simulink model "SG_GFOR_2020a_REAL"  (R2020a)
settings: Solver=ode1  StartTime=0.0  StopTime=Tsim  FixedStep=Ts  MaxStep=1e-4  RelTol=1e-4  EnableMultiTasking=on
values from neighbouring files (symbols this model uses):
  Cac_n1 = 1/5.88*(1/(w_n1*Xn_n1))    (= 2.64327804614e-06)    [VSC_GF_SG_params.m]
  f1 = 50    [VSC_GF_SG_params.m]
  f_n1 = f1    (= 50)    [VSC_GF_SG_params.m]
  k_droop_f_n1 = 1/20    (= 0.05)    [VSC_GF_SG_params.m]
  k_droop_u_n1 = 1e-4    (= 0.0001)    [VSC_GF_SG_params.m]
  ki_pll1 = kp_pll1/tau_pll_n1    [VSC_GF_SG_params.m]
  ki_s_n1 = Rc_n1/taus    (= 2048)    [VSC_GF_SG_params.m]
  ki_vac_n1 = 0.5    [VSC_GF_SG_params.m]
  kp_pll1 = xi_pll_n1*2*omega_pll_n1/Vpeak    [VSC_GF_SG_params.m]
  kp_s_n1 = Lc_n1/taus    (= 130.379729381)    [VSC_GF_SG_params.m]
  kp_vac_n1 = 0.025    [VSC_GF_SG_params.m]
  Lac = Lpu*l*(Un1/Vl)^2    (= 0.105785123967)    [VSC_GF_SG_params.m]
  Lc_n1 = 0.2*Ln_n1    (= 0.130379729381)    [VSC_GF_SG_params.m]
  magnitud_delay = Ts    (= 5e-05)    [VSC_GF_SG_params.m]
  Pload_fnl = 400e6    (= 400000000)    [VSC_GF_SG_params.m]
  plots_step = Ts    (= 5e-05)    [VSC_GF_SG_params.m]
  Pvsc0 = Pload0 -Psg0    (= 200000000)    [VSC_GF_SG_params.m]
  Q_ref_n1 = 10e6    (= 10000000)    [VSC_GF_SG_params.m]
  Rac = Rpu*l*(Un1/Vl)^2    (= 3.17355371901)    [VSC_GF_SG_params.m]
  Rc_n1 = 0.01*Xn_n1    (= 2.048)    [VSC_GF_SG_params.m]
  Rf = Rf_pu*Zfbase    [VSC_GF_SG_params.m]
  Sn1 = 500e6    (= 500000000)    [VSC_GF_SG_params.m]
  Sn_n2 = Sn1    (= 500000000)    [VSC_GF_SG_params.m]
  Ssg = 500e6    (= 500000000)    [VSC_GF_SG_params.m]
  T_stp = 20    [VSC_GF_SG_params.m]
  tau_droop_f = 0.1    [VSC_GF_SG_params.m]
  tau_droop_u = 40e-3    (= 0.04)    [VSC_GF_SG_params.m]
  tau_ig = 40e-3    (= 0.04)    [VSC_GF_SG_params.m]
  tau_u = 40e-3    (= 0.04)    [VSC_GF_SG_params.m]
  Ts = 5e-5    (= 5e-05)    [VSC_GF_SG_params.m]
  Un1 = 320e3    (= 320000)    [VSC_GF_SG_params.m]
  Vdcref_n1 = 640e3    (= 640000)    [VSC_GF_SG_params.m]
  Vpeak_n1 = Un_n1/sqrt(3)*sqrt(2)    [VSC_GF_SG_params.m]
  w_n1 = 2*pi*f_n1    (= 314.159265359)    [VSC_GF_SG_params.m]
undefined symbols (not defined in the file or in its folder): D11, Delta, Lf, P_set, P_step, Pload_init, Q_set, Q_step, t_ramp, t_step_P, t_step_Q, tau_ramp, tau_wf
libraries: powerlib x39, simulink x7, simulink_extras x6, powerlib_meascontrol x2
(part 2 of 2)

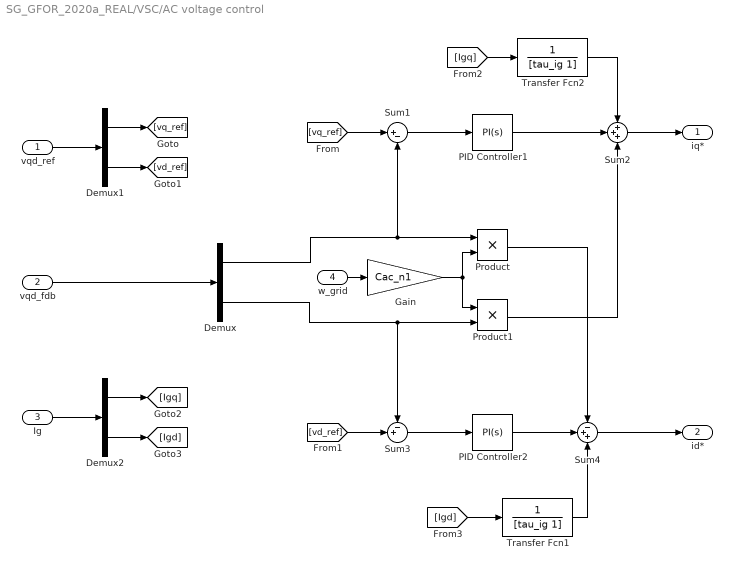
== system SG_GFOR_2020a_REAL/VSC/AC voltage control ==
  vqd_ref : Inport
  vqd_fdb : Inport  Port=2
  Ig : Inport  Port=3
  w_grid : Inport  Port=4
  Demux : Demux  Outputs=2
  Demux1 : Demux  Outputs=2
  Demux2 : Demux  Outputs=2
  Gain : Gain  Gain=Cac_n1
  PID Controller1 : simulink/Continuous/PID Controller  Controller=PI  Form=Parallel  TimeDomain=Continuous-time  UseExternalTs=off  SampleTime=-1  IntegratorMethod=Forward Euler  FilterMethod=Forward Euler  ControllerParametersSource=internal  P=kp_vac_n1  I=ki_vac_n1  D=0  UseFilter=on  N=100  TunerSelectOption=Transfer Function Based (PID Tuner App)  InitialConditionSource=internal  InitialConditionForIntegrator=0  InitialConditionForFilter=0  DifferentiatorICPrevScaledInput=0  ExternalReset=none  TrackingMode=off  Kt=1  LimitOutput=off  UpperSaturationLimit=inf  LowerSaturationLimit=-inf  LinearizeAsGain=on  AntiWindupMode=none  Kb=1  POutMin=[]  POutMax=[]  IOutMin=[]  IOutMax=[]  DOutMin=[]  DOutMax=[]  NOutMin=[]  NOutMax=[]  SumOutMin=[]  SumOutMax=[]  SaturationOutMin=[]  SaturationOutMax=[]  PParamMin=[]  PParamMax=[]  IParamMin=[]  IParamMax=[]  DParamMin=[]  DParamMax=[]  NParamMin=[]  NParamMax=[]  KbParamMin=[]  KbParamMax=[]  KtParamMin=[]  KtParamMax=[]  KbOutMin=[]  KbOutMax=[]  KtOutMin=[]  KtOutMax=[]  IntegratorOutMin=[]  IntegratorOutMax=[]  FilterOutMin=[]  FilterOutMax=[]  SumI1OutMin=[]  SumI1OutMax=[]  SumI2OutMin=[]  SumI2OutMax=[]  SumI3OutMin=[]  SumI3OutMax=[]  SumI4OutMin=[]  SumI4OutMax=[]  SumDOutMin=[]  SumDOutMax=[]  DifferentiatorOutMin=[]  DifferentiatorOutMax=[]  FilterDiffOutCoefMin=[]  FilterDiffOutCoefMax=[]  ReciprocalOutMin=[]  ReciprocalOutMax=[]  SumDenOutMin=[]  SumDenOutMax=[]  SumNumOutMin=[]  SumNumOutMax=[]  DivideOutMin=[]  DivideOutMax=[]  UdiffTsProdOutMin=[]  UdiffTsProdOutMax=[]  NTsProdOutMin=[]  NTsProdOutMax=[]  UintegralTsProdOutMin=[]  UintegralTsProdOutMax=[]  UngainTsProdOutMin=[]  UngainTsProdOutMax=[]  IntegratorContinuousStateAttributes=''  IntegratorStateMustResolveToSignalObject=off  IntegratorRTWStateStorageClass=Auto  FilterContinuousStateAttributes=''  FilterStateMustResolveToSignalObject=off  FilterRTWStateStorageClass=Auto  ParallelPVariant=InternalParameters  IdealPVariant=Disabled  IVariant=InternalParameters  DVariant=Disabled  IntegratorVariant=Continuous  SatVariant=Disabled  AWVariant=Passthrough  PCopyVariant=Disabled  TRVariant=Disabled  FdbkBlocksVariant=Forward  IdealPFdbkVariant=Disabled  SatFdbkVariant=Disabled  DerivativeFilterVariant=Disabled  NVariant=Disabled  NCopyVariant=Disabled_SignalSpec  FilterICVariant=Disabled  IntegratorICVariant=InternalICs  ExternalResetVariant=Disabled  TRSumVariant=Passthrough  SumFdbkVariant=Disabled  SumVariant=Sum_PI  TsampFilterVariant=InternalTs  TsampNgainVariant=Passthrough  TsampIntegralVariant=Passthrough
  PID Controller2 : simulink/Continuous/PID Controller  Controller=PI  Form=Parallel  TimeDomain=Continuous-time  UseExternalTs=off  SampleTime=-1  IntegratorMethod=Forward Euler  FilterMethod=Forward Euler  ControllerParametersSource=internal  P=kp_vac_n1  I=ki_vac_n1  D=0  UseFilter=on  N=100  TunerSelectOption=Transfer Function Based (PID Tuner App)  InitialConditionSource=internal  InitialConditionForIntegrator=0  InitialConditionForFilter=0  DifferentiatorICPrevScaledInput=0  ExternalReset=none  TrackingMode=off  Kt=1  LimitOutput=off  UpperSaturationLimit=inf  LowerSaturationLimit=-inf  LinearizeAsGain=on  AntiWindupMode=none  Kb=1  POutMin=[]  POutMax=[]  IOutMin=[]  IOutMax=[]  DOutMin=[]  DOutMax=[]  NOutMin=[]  NOutMax=[]  SumOutMin=[]  SumOutMax=[]  SaturationOutMin=[]  SaturationOutMax=[]  PParamMin=[]  PParamMax=[]  IParamMin=[]  IParamMax=[]  DParamMin=[]  DParamMax=[]  NParamMin=[]  NParamMax=[]  KbParamMin=[]  KbParamMax=[]  KtParamMin=[]  KtParamMax=[]  KbOutMin=[]  KbOutMax=[]  KtOutMin=[]  KtOutMax=[]  IntegratorOutMin=[]  IntegratorOutMax=[]  FilterOutMin=[]  FilterOutMax=[]  SumI1OutMin=[]  SumI1OutMax=[]  SumI2OutMin=[]  SumI2OutMax=[]  SumI3OutMin=[]  SumI3OutMax=[]  SumI4OutMin=[]  SumI4OutMax=[]  SumDOutMin=[]  SumDOutMax=[]  DifferentiatorOutMin=[]  DifferentiatorOutMax=[]  FilterDiffOutCoefMin=[]  FilterDiffOutCoefMax=[]  ReciprocalOutMin=[]  ReciprocalOutMax=[]  SumDenOutMin=[]  SumDenOutMax=[]  SumNumOutMin=[]  SumNumOutMax=[]  DivideOutMin=[]  DivideOutMax=[]  UdiffTsProdOutMin=[]  UdiffTsProdOutMax=[]  NTsProdOutMin=[]  NTsProdOutMax=[]  UintegralTsProdOutMin=[]  UintegralTsProdOutMax=[]  UngainTsProdOutMin=[]  UngainTsProdOutMax=[]  IntegratorContinuousStateAttributes=''  IntegratorStateMustResolveToSignalObject=off  IntegratorRTWStateStorageClass=Auto  FilterContinuousStateAttributes=''  FilterStateMustResolveToSignalObject=off  FilterRTWStateStorageClass=Auto  ParallelPVariant=InternalParameters  IdealPVariant=Disabled  IVariant=InternalParameters  DVariant=Disabled  IntegratorVariant=Continuous  SatVariant=Disabled  AWVariant=Passthrough  PCopyVariant=Disabled  TRVariant=Disabled  FdbkBlocksVariant=Forward  IdealPFdbkVariant=Disabled  SatFdbkVariant=Disabled  DerivativeFilterVariant=Disabled  NVariant=Disabled  NCopyVariant=Disabled_SignalSpec  FilterICVariant=Disabled  IntegratorICVariant=InternalICs  ExternalResetVariant=Disabled  TRSumVariant=Passthrough  SumFdbkVariant=Disabled  SumVariant=Sum_PI  TsampFilterVariant=InternalTs  TsampNgainVariant=Passthrough  TsampIntegralVariant=Passthrough
  Product : Product  RndMeth=Zero
  Product1 : Product  RndMeth=Zero
  Sum1 : Sum  Inputs=|+-
  Sum2 : Sum  Inputs=+++
  Sum3 : Sum  Inputs=-+|
  Sum4 : Sum  Inputs=-++
  Transfer Fcn1 : TransferFcn  Denominator=[tau_ig 1]
  Transfer Fcn2 : TransferFcn  Denominator=[tau_ig 1]
  iq* : Outport
  id* : Outport  Port=2
  wires:
  Ig/1 -> Demux2/1
  Demux2/2 -> [Igd]
  Demux2/1 -> [Igq]
  Demux1/2 -> [vd_ref]
  Demux1/1 -> [vq_ref]
  vqd_ref/1 -> Demux1/1
  [vd_ref] -> Sum3/2
  Product/1 -> Sum4/1
  Product1/1 -> Sum2/3
  Demux/2 -> Sum3/1, Product1/2
  Sum3/1 -> PID Controller2/1
  Gain/1 -> Product/2, Product1/1
  Demux/1 -> Product/1, Sum1/2
  PID Controller1/1 -> Sum2/2
  w_grid/1 -> Gain/1
  [vq_ref] -> Sum1/1
  Sum1/1 -> PID Controller1/1
  vqd_fdb/1 -> Demux/1
  [Igq] -> Transfer Fcn2/1
  [Igd] -> Transfer Fcn1/1
  Sum2/1 -> iq*/1
  Sum4/1 -> id*/1
  PID Controller2/1 -> Sum4/2
  Transfer Fcn2/1 -> Sum2/1
  Transfer Fcn1/1 -> Sum4/3

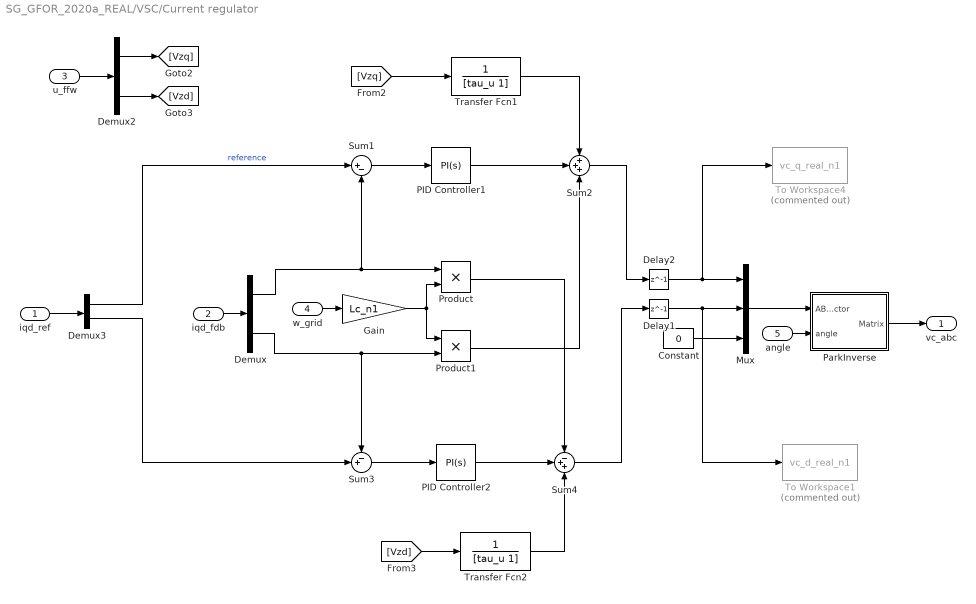
== system SG_GFOR_2020a_REAL/VSC/Current regulator ==
  iqd_ref : Inport
  iqd_fdb : Inport  Port=2
  u_ffw : Inport  Port=3
  w_grid : Inport  Port=4
  angle : Inport  Port=5
  Constant : Constant  Value=0
  Delay1 : Delay  DelayLength=1  InitialCondition=0  SampleTime=magnitud_delay
  Delay2 : Delay  DelayLength=1  InitialCondition=Vpeak_n1  SampleTime=magnitud_delay
  Demux : Demux  Outputs=2
  Demux2 : Demux  Outputs=2
  Demux3 : Demux  Outputs=2
  Gain : Gain  Gain=Lc_n1
  Mux : Mux  Inputs=3
  PID Controller1 : simulink/Continuous/PID Controller  Controller=PI  Form=Parallel  TimeDomain=Continuous-time  UseExternalTs=off  SampleTime=-1  IntegratorMethod=Forward Euler  FilterMethod=Forward Euler  ControllerParametersSource=internal  P=kp_s_n1  I=ki_s_n1  D=0  UseFilter=on  N=100  TunerSelectOption=Transfer Function Based (PID Tuner App)  InitialConditionSource=internal  InitialConditionForIntegrator=0  InitialConditionForFilter=0  DifferentiatorICPrevScaledInput=0  ExternalReset=none  TrackingMode=off  Kt=1  LimitOutput=off  UpperSaturationLimit=inf  LowerSaturationLimit=-inf  LinearizeAsGain=on  AntiWindupMode=none  Kb=1  POutMin=[]  POutMax=[]  IOutMin=[]  IOutMax=[]  DOutMin=[]  DOutMax=[]  NOutMin=[]  NOutMax=[]  SumOutMin=[]  SumOutMax=[]  SaturationOutMin=[]  SaturationOutMax=[]  PParamMin=[]  PParamMax=[]  IParamMin=[]  IParamMax=[]  DParamMin=[]  DParamMax=[]  NParamMin=[]  NParamMax=[]  KbParamMin=[]  KbParamMax=[]  KtParamMin=[]  KtParamMax=[]  KbOutMin=[]  KbOutMax=[]  KtOutMin=[]  KtOutMax=[]  IntegratorOutMin=[]  IntegratorOutMax=[]  FilterOutMin=[]  FilterOutMax=[]  SumI1OutMin=[]  SumI1OutMax=[]  SumI2OutMin=[]  SumI2OutMax=[]  SumI3OutMin=[]  SumI3OutMax=[]  SumI4OutMin=[]  SumI4OutMax=[]  SumDOutMin=[]  SumDOutMax=[]  DifferentiatorOutMin=[]  DifferentiatorOutMax=[]  FilterDiffOutCoefMin=[]  FilterDiffOutCoefMax=[]  ReciprocalOutMin=[]  ReciprocalOutMax=[]  SumDenOutMin=[]  SumDenOutMax=[]  SumNumOutMin=[]  SumNumOutMax=[]  DivideOutMin=[]  DivideOutMax=[]  UdiffTsProdOutMin=[]  UdiffTsProdOutMax=[]  NTsProdOutMin=[]  NTsProdOutMax=[]  UintegralTsProdOutMin=[]  UintegralTsProdOutMax=[]  UngainTsProdOutMin=[]  UngainTsProdOutMax=[]  IntegratorContinuousStateAttributes=''  IntegratorStateMustResolveToSignalObject=off  IntegratorRTWStateStorageClass=Auto  FilterContinuousStateAttributes=''  FilterStateMustResolveToSignalObject=off  FilterRTWStateStorageClass=Auto  ParallelPVariant=InternalParameters  IdealPVariant=Disabled  IVariant=InternalParameters  DVariant=Disabled  IntegratorVariant=Continuous  SatVariant=Disabled  AWVariant=Passthrough  PCopyVariant=Disabled  TRVariant=Disabled  FdbkBlocksVariant=Forward  IdealPFdbkVariant=Disabled  SatFdbkVariant=Disabled  DerivativeFilterVariant=Disabled  NVariant=Disabled  NCopyVariant=Disabled_SignalSpec  FilterICVariant=Disabled  IntegratorICVariant=InternalICs  ExternalResetVariant=Disabled  TRSumVariant=Passthrough  SumFdbkVariant=Disabled  SumVariant=Sum_PI  TsampFilterVariant=InternalTs  TsampNgainVariant=Passthrough  TsampIntegralVariant=Passthrough
  PID Controller2 : simulink/Continuous/PID Controller  Controller=PI  Form=Parallel  TimeDomain=Continuous-time  UseExternalTs=off  SampleTime=-1  IntegratorMethod=Forward Euler  FilterMethod=Forward Euler  ControllerParametersSource=internal  P=kp_s_n1  I=ki_s_n1  D=0  UseFilter=on  N=100  TunerSelectOption=Transfer Function Based (PID Tuner App)  InitialConditionSource=internal  InitialConditionForIntegrator=0  InitialConditionForFilter=0  DifferentiatorICPrevScaledInput=0  ExternalReset=none  TrackingMode=off  Kt=1  LimitOutput=off  UpperSaturationLimit=inf  LowerSaturationLimit=-inf  LinearizeAsGain=on  AntiWindupMode=none  Kb=1  POutMin=[]  POutMax=[]  IOutMin=[]  IOutMax=[]  DOutMin=[]  DOutMax=[]  NOutMin=[]  NOutMax=[]  SumOutMin=[]  SumOutMax=[]  SaturationOutMin=[]  SaturationOutMax=[]  PParamMin=[]  PParamMax=[]  IParamMin=[]  IParamMax=[]  DParamMin=[]  DParamMax=[]  NParamMin=[]  NParamMax=[]  KbParamMin=[]  KbParamMax=[]  KtParamMin=[]  KtParamMax=[]  KbOutMin=[]  KbOutMax=[]  KtOutMin=[]  KtOutMax=[]  IntegratorOutMin=[]  IntegratorOutMax=[]  FilterOutMin=[]  FilterOutMax=[]  SumI1OutMin=[]  SumI1OutMax=[]  SumI2OutMin=[]  SumI2OutMax=[]  SumI3OutMin=[]  SumI3OutMax=[]  SumI4OutMin=[]  SumI4OutMax=[]  SumDOutMin=[]  SumDOutMax=[]  DifferentiatorOutMin=[]  DifferentiatorOutMax=[]  FilterDiffOutCoefMin=[]  FilterDiffOutCoefMax=[]  ReciprocalOutMin=[]  ReciprocalOutMax=[]  SumDenOutMin=[]  SumDenOutMax=[]  SumNumOutMin=[]  SumNumOutMax=[]  DivideOutMin=[]  DivideOutMax=[]  UdiffTsProdOutMin=[]  UdiffTsProdOutMax=[]  NTsProdOutMin=[]  NTsProdOutMax=[]  UintegralTsProdOutMin=[]  UintegralTsProdOutMax=[]  UngainTsProdOutMin=[]  UngainTsProdOutMax=[]  IntegratorContinuousStateAttributes=''  IntegratorStateMustResolveToSignalObject=off  IntegratorRTWStateStorageClass=Auto  FilterContinuousStateAttributes=''  FilterStateMustResolveToSignalObject=off  FilterRTWStateStorageClass=Auto  ParallelPVariant=InternalParameters  IdealPVariant=Disabled  IVariant=InternalParameters  DVariant=Disabled  IntegratorVariant=Continuous  SatVariant=Disabled  AWVariant=Passthrough  PCopyVariant=Disabled  TRVariant=Disabled  FdbkBlocksVariant=Forward  IdealPFdbkVariant=Disabled  SatFdbkVariant=Disabled  DerivativeFilterVariant=Disabled  NVariant=Disabled  NCopyVariant=Disabled_SignalSpec  FilterICVariant=Disabled  IntegratorICVariant=InternalICs  ExternalResetVariant=Disabled  TRSumVariant=Passthrough  SumFdbkVariant=Disabled  SumVariant=Sum_PI  TsampFilterVariant=InternalTs  TsampNgainVariant=Passthrough  TsampIntegralVariant=Passthrough
  ParkInverse : Subsystem  mask(Gerard){}
      mask help:
      | This block applies the park inverse transfomation from a desired vector.
      | The input Xqd0 refers to the vector in the qd0 frame, and the second input is the angle used in the inverse transformation.
      | The output is the vector in the ABC frame.
      mask Display:
      | port_label('output',1,'Xabc')
      | port_label('input',1,'Xqd0')
      | port_label('input',2,'angle')
  Product : Product  RndMeth=Zero
  Product1 : Product  RndMeth=Zero
  Sum1 : Sum  Inputs=|+-
  Sum2 : Sum  Inputs=+++
  Sum3 : Sum  Inputs=-+|
  Sum4 : Sum  Inputs=-++
  To Workspace1 : ToWorkspace  Commented=on  VariableName=vc_d_real_n1  SampleTime=plots_step
  To Workspace4 : ToWorkspace  Commented=on  VariableName=vc_q_real_n1  SampleTime=plots_step
  Transfer Fcn1 : TransferFcn  Denominator=[tau_u 1]
  Transfer Fcn2 : TransferFcn  Denominator=[tau_u 1]
  vc_abc : Outport
  wires:
  iqd_fdb/1 -> Demux/1
  w_grid/1 -> Gain/1
  PID Controller1/1 -> Sum2/2
  Demux/1 -> Sum1/2, Product/1
  Gain/1 -> Product1/1, Product/2
  Demux/2 -> Product1/2, Sum3/1
  Product1/1 -> Sum2/3
  Product/1 -> Sum4/1
  Constant/1 -> Mux/3
  ParkInverse/1(Matrix) -> vc_abc/1
  Transfer Fcn1/1 -> Sum2/1
  Mux/1 -> ParkInverse/1(ABC vector)
  Demux2/1 -> [Vzq]
  Demux2/2 -> [Vzd]
  u_ffw/1 -> Demux2/1
  [Vzd] -> Transfer Fcn2/1
  angle/1 -> ParkInverse/2(angle)
  Sum1/1 -> PID Controller1/1
  Sum3/1 -> PID Controller2/1
  PID Controller2/1 -> Sum4/2
  Demux3/1 -> Sum1/1  "reference"
  iqd_ref/1 -> Demux3/1
  Sum2/1 -> Delay2/1
  Sum4/1 -> Delay1/1
  Demux3/2 -> Sum3/2
  [Vzq] -> Transfer Fcn1/1
  Transfer Fcn2/1 -> Sum4/3
  Delay2/1 -> To Workspace4/1, Mux/1
  Delay1/1 -> Mux/2, To Workspace1/1

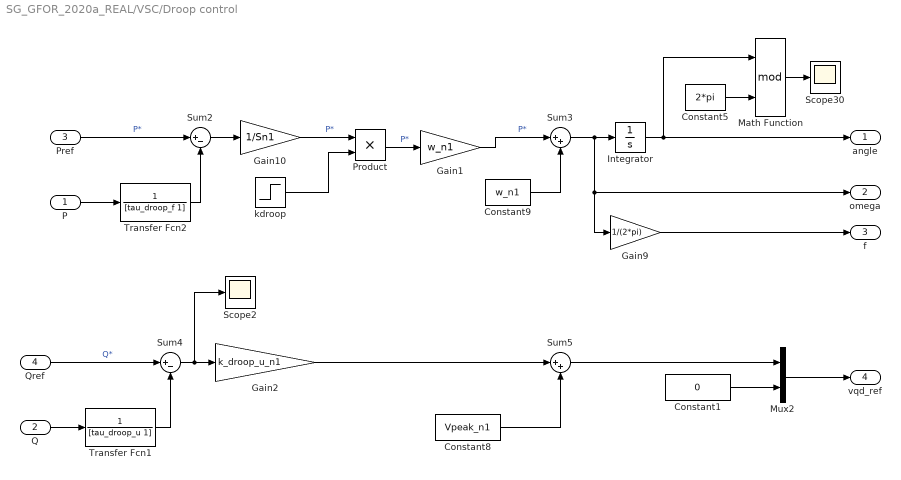
== system SG_GFOR_2020a_REAL/VSC/Droop control ==
  P : Inport
  Q : Inport  Port=2
  Pref : Inport  Port=3
  Qref : Inport  Port=4
  Constant1 : Constant  Value=0
  Constant5 : Constant  Value=2*pi
  Constant8 : Constant  Value=Vpeak_n1
  Constant9 : Constant  Value=w_n1
  Gain1 : Gain  Gain=w_n1
  Gain10 : Gain  Gain=1/Sn1
  Gain2 : Gain  Gain=k_droop_u_n1
  Gain9 : Gain  Gain=1/(2*pi)
  Integrator : Integrator
  Math Function : Math  Operator=mod  SignedPower=on  SaturateOnIntegerOverflow=on
  Mux2 : Mux  Inputs=2
  Product : Product
  Scope2 : Scope
  Scope30 : Scope
  Sum2 : Sum  Inputs=|+-
  Sum3 : Sum  Inputs=|++
  Sum4 : Sum  Inputs=|+-
  Sum5 : Sum  Inputs=|++
  Transfer Fcn1 : TransferFcn  Denominator=[tau_droop_u 1]
  Transfer Fcn2 : TransferFcn  Denominator=[tau_droop_f 1]
  kdroop : Step  Time=100  Before=k_droop_f_n1  After=k_droop_f_n1  SampleTime=0
  angle : Outport
  omega : Outport  Port=2
  f : Outport  Port=3
  vqd_ref : Outport  Port=4
  wires:
  Gain9/1 -> f/1
  Pref/1 -> Sum2/1  "P*"
  Sum2/1 -> Gain10/1
  Integrator/1 -> angle/1, Math Function/1
  Constant9/1 -> Sum3/2
  Sum3/1 -> omega/1, Gain9/1, Integrator/1
  Math Function/1 -> Scope30/1
  P/1 -> Transfer Fcn2/1
  Constant5/1 -> Math Function/2
  Transfer Fcn1/1 -> Sum4/2
  Qref/1 -> Sum4/1  "Q*"
  Q/1 -> Transfer Fcn1/1
  Sum4/1 -> Scope2/1, Gain2/1
  Sum5/1 -> Mux2/1
  Mux2/1 -> vqd_ref/1
  Constant1/1 -> Mux2/2
  Constant8/1 -> Sum5/2
  Product/1 -> Gain1/1  "P*"
  Gain2/1 -> Sum5/1
  kdroop/1 -> Product/2
  Transfer Fcn2/1 -> Sum2/2
  Gain10/1 -> Product/1  "P*"
  Gain1/1 -> Sum3/1  "P*"

== system SG_GFOR_2020a_REAL/VSC/PQ Calculation1 ==
  u_qd : Inport
  ig_qd : Inport  Port=2
  Add1 : Sum  Inputs=-+
  Add2 : Sum
  Demux4 : Demux  Outputs=2
  Demux7 : Demux  Outputs=2
  Gain1 : Gain  Gain=3/2
  Gain12 : Gain  Gain=3/2
  Product{,1..3} (4 alike) : Product
  P : Outport
  Q : Outport  Port=2
  wires:
  Demux4/2 -> Product1/2, Product3/2
  Demux7/2 -> Product2/1, Product1/1
  Product/1 -> Add2/1
  Product1/1 -> Add2/2
  Add2/1 -> Gain12/1
  Demux7/1 -> Product3/1, Product/1
  Product2/1 -> Add1/1
  Demux4/1 -> Product2/2, Product/2
  Add1/1 -> Gain1/1
  Product3/1 -> Add1/2
  ig_qd/1 -> Demux4/1
  u_qd/1 -> Demux7/1
  Gain1/1 -> Q/1
  Gain12/1 -> P/1

== system SG_GFOR_2020a_REAL/VSC/ParkTransform2 ==
  ABC vector : Inport
  angle : Inport  Port=2
  Constant1 : Constant  Value=1/2
  Constant2 : Constant  Value=1/2
  Constant3 : Constant  Value=2*pi/3
  Constant4 : Constant  Value=2*pi/3
  Constant5 : Constant  Value=1/2
  Gain : Gain  Gain=2/3
  Matrix Concatenate : Concatenate  NumInputs=3  Mode=Multidimensional array  ConcatenateDimension=2
  Mux1 : Mux  Inputs=3
  Mux2 : Mux  Inputs=3
  Mux3 : Mux  Inputs=3
  Product : Product  Multiplication=Matrix(*)  RndMeth=Zero
  Sum : Sum  Inputs=|+-
  Sum1 : Sum  Inputs=|++
  Trigonometric Function1 : Trigonometry  Operator=cos
  Trigonometric Function2 : Trigonometry  Operator=cos
  Trigonometric Function3 : Trigonometry
  Trigonometric Function4 : Trigonometry
  Trigonometric Function5 : Trigonometry  Operator=cos
  Trigonometric Function6 : Trigonometry
  Matrix : Outport
  wires:
  Matrix Concatenate/1 -> Gain/1
  ABC vector/1 -> Product/2
  Product/1 -> Matrix/1
  Gain/1 -> Product/1
  Constant4/1 -> Sum/2
  Constant3/1 -> Sum1/2
  angle/1 -> Trigonometric Function4/1, Trigonometric Function1/1, Sum1/1, Sum/1
  Trigonometric Function3/1 -> Mux1/2
  Trigonometric Function2/1 -> Mux1/1
  Constant2/1 -> Mux1/3
  Sum/1 -> Trigonometric Function3/1, Trigonometric Function2/1
  Trigonometric Function4/1 -> Mux2/2
  Trigonometric Function1/1 -> Mux2/1
  Constant1/1 -> Mux2/3
  Trigonometric Function6/1 -> Mux3/2
  Trigonometric Function5/1 -> Mux3/1
  Constant5/1 -> Mux3/3
  Sum1/1 -> Trigonometric Function6/1, Trigonometric Function5/1
  Mux1/1 -> Matrix Concatenate/2
  Mux2/1 -> Matrix Concatenate/1
  Mux3/1 -> Matrix Concatenate/3

== system SG_GFOR_2020a_REAL/VSC/ParkTransform3 ==
  ABC vector : Inport
  angle : Inport  Port=2
  Constant1 : Constant  Value=1/2
  Constant2 : Constant  Value=1/2
  Constant3 : Constant  Value=2*pi/3
  Constant4 : Constant  Value=2*pi/3
  Constant5 : Constant  Value=1/2
  Gain : Gain  Gain=2/3
  Matrix Concatenate : Concatenate  NumInputs=3  Mode=Multidimensional array  ConcatenateDimension=2
  Mux1 : Mux  Inputs=3
  Mux2 : Mux  Inputs=3
  Mux3 : Mux  Inputs=3
  Product : Product  Multiplication=Matrix(*)  RndMeth=Zero
  Sum : Sum  Inputs=|+-
  Sum1 : Sum  Inputs=|++
  Trigonometric Function1 : Trigonometry  Operator=cos
  Trigonometric Function2 : Trigonometry  Operator=cos
  Trigonometric Function3 : Trigonometry
  Trigonometric Function4 : Trigonometry
  Trigonometric Function5 : Trigonometry  Operator=cos
  Trigonometric Function6 : Trigonometry
  Matrix : Outport
  wires:
  Mux3/1 -> Matrix Concatenate/3
  Mux2/1 -> Matrix Concatenate/1
  Mux1/1 -> Matrix Concatenate/2
  Sum1/1 -> Trigonometric Function5/1, Trigonometric Function6/1
  Constant5/1 -> Mux3/3
  Trigonometric Function5/1 -> Mux3/1
  Trigonometric Function6/1 -> Mux3/2
  Constant1/1 -> Mux2/3
  Trigonometric Function1/1 -> Mux2/1
  Trigonometric Function4/1 -> Mux2/2
  Sum/1 -> Trigonometric Function2/1, Trigonometric Function3/1
  Constant2/1 -> Mux1/3
  Trigonometric Function2/1 -> Mux1/1
  Trigonometric Function3/1 -> Mux1/2
  angle/1 -> Sum/1, Sum1/1, Trigonometric Function1/1, Trigonometric Function4/1
  Constant3/1 -> Sum1/2
  Constant4/1 -> Sum/2
  Gain/1 -> Product/1
  Product/1 -> Matrix/1
  ABC vector/1 -> Product/2
  Matrix Concatenate/1 -> Gain/1

== system SG_GFOR_2020a_REAL/VSC/ParkTransform4 ==
  ABC vector : Inport
  angle : Inport  Port=2
  Constant1 : Constant  Value=1/2
  Constant2 : Constant  Value=1/2
  Constant3 : Constant  Value=2*pi/3
  Constant4 : Constant  Value=2*pi/3
  Constant5 : Constant  Value=1/2
  Gain : Gain  Gain=2/3
  Matrix Concatenate : Concatenate  NumInputs=3  Mode=Multidimensional array  ConcatenateDimension=2
  Mux1 : Mux  Inputs=3
  Mux2 : Mux  Inputs=3
  Mux3 : Mux  Inputs=3
  Product : Product  Multiplication=Matrix(*)  RndMeth=Zero
  Sum : Sum  Inputs=|+-
  Sum1 : Sum  Inputs=|++
  Trigonometric Function1 : Trigonometry  Operator=cos
  Trigonometric Function2 : Trigonometry  Operator=cos
  Trigonometric Function3 : Trigonometry
  Trigonometric Function4 : Trigonometry
  Trigonometric Function5 : Trigonometry  Operator=cos
  Trigonometric Function6 : Trigonometry
  Matrix : Outport
  wires:
  Mux3/1 -> Matrix Concatenate/3
  Mux2/1 -> Matrix Concatenate/1
  Mux1/1 -> Matrix Concatenate/2
  Sum1/1 -> Trigonometric Function5/1, Trigonometric Function6/1
  Constant5/1 -> Mux3/3
  Trigonometric Function5/1 -> Mux3/1
  Trigonometric Function6/1 -> Mux3/2
  Constant1/1 -> Mux2/3
  Trigonometric Function1/1 -> Mux2/1
  Trigonometric Function4/1 -> Mux2/2
  Sum/1 -> Trigonometric Function2/1, Trigonometric Function3/1
  Constant2/1 -> Mux1/3
  Trigonometric Function2/1 -> Mux1/1
  Trigonometric Function3/1 -> Mux1/2
  angle/1 -> Sum/1, Sum1/1, Trigonometric Function1/1, Trigonometric Function4/1
  Constant3/1 -> Sum1/2
  Constant4/1 -> Sum/2
  Gain/1 -> Product/1
  Product/1 -> Matrix/1
  ABC vector/1 -> Product/2
  Matrix Concatenate/1 -> Gain/1

== system SG_GFOR_2020a_REAL/VSC/VSC n1 ==
  vc_abc : Inport
  i_abc : Inport  Port=2
  Vbus : Inport  Port=3
  Controlled Current Source5 : powerlib/Electrical Sources/Controlled Current Source  Initialize=on  Source_Type=DC  Amplitude=0  Phase=0  Frequency=0  Measurements=None
  Controlled Voltage Source1 : powerlib/Electrical Sources/Controlled Voltage Source  Initialize=off  Source_Type=AC  Amplitude=0  Phase=0  Frequency=0  Measurements=None
  Controlled Voltage Source2 : powerlib/Electrical Sources/Controlled Voltage Source  Initialize=off  Source_Type=AC  Amplitude=0  Phase=0  Frequency=0  Measurements=None
  Controlled Voltage Source3 : powerlib/Electrical Sources/Controlled Voltage Source  Initialize=off  Source_Type=AC  Amplitude=0  Phase=0  Frequency=0  Measurements=None
  Current Measurement9 : powerlib/Measurements/Current Measurement  PhasorSimulation=off  OutputType=Complex  PSBequivalent=0
  Demux : Demux  Outputs=3
  Divide : Product  Inputs=*/
  Ground : powerlib/Elements/Ground  LConnTagsString=a
  Product1 : Product  InputSameDT=on  SaturateOnIntegerOverflow=on  OutDataTypeStr=Inherit: Same as first input
  Sum4 : Sum  Inputs=1  InputSameDT=on  SaturateOnIntegerOverflow=on  OutDataTypeStr=Inherit: Same as first input
  vc_abc1 : InportShadow
  a : PMIOPort  Side=Left
  b : PMIOPort  Port=2  Side=Left
  c : PMIOPort  Port=3  Side=Left
  DC+ : PMIOPort  Port=4  Side=Right
  DC- : PMIOPort  Port=5  Side=Right
  idc : Outport
  wires:
  Current Measurement9/1 -> idc/1
  Product1/1 -> Sum4/1
  Sum4/1 -> Divide/1
  Divide/1 -> Controlled Current Source5/1
  vc_abc1/1 -> Product1/1
  i_abc/1 -> Product1/2
  Demux/2 -> Controlled Voltage Source2/1
  Demux/1 -> Controlled Voltage Source1/1
  Demux/3 -> Controlled Voltage Source3/1
  vc_abc/1 -> Demux/1
  Vbus/1 -> Divide/2
  connections:
  Controlled Current Source5/RConn1 -- DC-/RConn1
  Controlled Current Source5/LConn1 -- Current Measurement9/RConn1
  Current Measurement9/LConn1 -- DC+/RConn1
  Controlled Voltage Source1/LConn1 -- Controlled Voltage Source2/LConn1 -- Ground/LConn1 -- Controlled Voltage Source3/LConn1
  a/RConn1 -- Controlled Voltage Source1/RConn1
  b/RConn1 -- Controlled Voltage Source2/RConn1
  c/RConn1 -- Controlled Voltage Source3/RConn1

== system SG_GFOR_2020a_REAL/Do not use/PQ/PLL ==
  u_abc : Inport
  Constant : Constant  Value=0
  Constant3 : Constant  Value=2*pi*f_n1
  Constant4 : Constant  Value=2*pi
  Demux : Demux  Outputs=3
  Integrator : Integrator
  Math Function : Math  Operator=mod  SignedPower=on  SaturateOnIntegerOverflow=on
  PID Controller : simulink/Continuous/PID Controller  Controller=PI  Form=Parallel  TimeDomain=Continuous-time  UseExternalTs=off  SampleTime=-1  IntegratorMethod=Forward Euler  FilterMethod=Forward Euler  ControllerParametersSource=internal  P=kp_pll1  I=ki_pll1  D=0  UseFilter=on  N=100  TunerSelectOption=Transfer Function Based (PID Tuner App)  InitialConditionSource=internal  InitialConditionForIntegrator=0  InitialConditionForFilter=0  DifferentiatorICPrevScaledInput=0  ExternalReset=none  TrackingMode=off  Kt=1  LimitOutput=off  UpperSaturationLimit=inf  LowerSaturationLimit=-inf  LinearizeAsGain=on  AntiWindupMode=none  Kb=1  POutMin=[]  POutMax=[]  IOutMin=[]  IOutMax=[]  DOutMin=[]  DOutMax=[]  NOutMin=[]  NOutMax=[]  SumOutMin=[]  SumOutMax=[]  SaturationOutMin=[]  SaturationOutMax=[]  PParamMin=[]  PParamMax=[]  IParamMin=[]  IParamMax=[]  DParamMin=[]  DParamMax=[]  NParamMin=[]  NParamMax=[]  KbParamMin=[]  KbParamMax=[]  KtParamMin=[]  KtParamMax=[]  KbOutMin=[]  KbOutMax=[]  KtOutMin=[]  KtOutMax=[]  IntegratorOutMin=[]  IntegratorOutMax=[]  FilterOutMin=[]  FilterOutMax=[]  SumI1OutMin=[]  SumI1OutMax=[]  SumI2OutMin=[]  SumI2OutMax=[]  SumI3OutMin=[]  SumI3OutMax=[]  SumI4OutMin=[]  SumI4OutMax=[]  SumDOutMin=[]  SumDOutMax=[]  DifferentiatorOutMin=[]  DifferentiatorOutMax=[]  FilterDiffOutCoefMin=[]  FilterDiffOutCoefMax=[]  ReciprocalOutMin=[]  ReciprocalOutMax=[]  SumDenOutMin=[]  SumDenOutMax=[]  SumNumOutMin=[]  SumNumOutMax=[]  DivideOutMin=[]  DivideOutMax=[]  UdiffTsProdOutMin=[]  UdiffTsProdOutMax=[]  NTsProdOutMin=[]  NTsProdOutMax=[]  UintegralTsProdOutMin=[]  UintegralTsProdOutMax=[]  UngainTsProdOutMin=[]  UngainTsProdOutMax=[]  IntegratorContinuousStateAttributes=''  IntegratorStateMustResolveToSignalObject=off  IntegratorRTWStateStorageClass=Auto  FilterContinuousStateAttributes=''  FilterStateMustResolveToSignalObject=off  FilterRTWStateStorageClass=Auto  ParallelPVariant=InternalParameters  IdealPVariant=Disabled  IVariant=InternalParameters  DVariant=Disabled  IntegratorVariant=Continuous  SatVariant=Disabled  AWVariant=Passthrough  PCopyVariant=Disabled  TRVariant=Disabled  FdbkBlocksVariant=Forward  IdealPFdbkVariant=Disabled  SatFdbkVariant=Disabled  DerivativeFilterVariant=Disabled  NVariant=Disabled  NCopyVariant=Disabled_SignalSpec  FilterICVariant=Disabled  IntegratorICVariant=InternalICs  ExternalResetVariant=Disabled  TRSumVariant=Passthrough  SumFdbkVariant=Disabled  SumVariant=Sum_PI  TsampFilterVariant=InternalTs  TsampNgainVariant=Passthrough  TsampIntegralVariant=Passthrough
  ParkTransform7 : Subsystem  mask(Gerard){}
      mask help:
      | This block applies the park transfomation from a desired vector.
      | The input Xabc refers to the vector in the ABC frame, and the second input is the angle used in the transformation.
      | The output is the vector in the qd0 frame.
      mask Display:
      | port_label('output',1,'Xqd0')
      | port_label('input',1,'Xabc')
      | port_label('input',2,'angle')
  Scope1 : Scope
  Scope20 : Scope
  Sum : Sum  Inputs=|+-
  Sum1 : Sum  Inputs=|++
  Terminator8 : Terminator
  Vzq : Outport
  Vzd : Outport  Port=2
  angle : Outport  Port=3
  w_grid : Outport  Port=4
  wires:
  Math Function/1 -> Scope1/1
  Demux/1 -> Vzq/1
  Sum/1 -> PID Controller/1, Scope20/1
  ParkTransform7/1(Matrix) -> Demux/1
  u_abc/1 -> ParkTransform7/1(ABC vector)
  PID Controller/1 -> Sum1/1
  Demux/3 -> Terminator8/1
  Integrator/1 -> angle/1, Math Function/1, ParkTransform7/2(angle)
  Constant4/1 -> Math Function/2
  Constant/1 -> Sum/1
  Sum1/1 -> Integrator/1, w_grid/1
  Demux/2 -> Sum/2, Vzd/1
  Constant3/1 -> Sum1/2

== system SG_GFOR_2020a_REAL/Do not use/PQ/ParkInverse1 ==
  ABC vector : Inport
  angle : Inport  Port=2
  Constant4 : Constant  Value=2*pi/3
  Constant5 : Constant  Value=2*pi/3
  Constant9 : Constant
  Matrix Concatenate2 : Concatenate  NumInputs=3  Mode=Multidimensional array  ConcatenateDimension=2
  Mux6 : Mux  Inputs=3
  Mux7 : Mux  Inputs=3
  Product : Product  Multiplication=Matrix(*)  RndMeth=Zero
  Signal Specification1 : SignalSpecification  Dimensions=3
  Signal Specification4 : SignalSpecification  Dimensions=3
  Sum : Sum  Inputs=|+-
  Sum1 : Sum  Inputs=|++
  Trigonometric Function8 : Trigonometry  Operator=cos
  Trigonometric Function9 : Trigonometry
  Matrix : Outport
  wires:
  Signal Specification1/1 -> Matrix Concatenate2/2
  Signal Specification4/1 -> Matrix Concatenate2/1
  angle/1 -> Sum1/1, Sum/1, Mux6/1
  Constant5/1 -> Sum1/2
  Constant4/1 -> Sum/2
  Product/1 -> Matrix/1
  ABC vector/1 -> Product/2
  Sum/1 -> Mux6/2
  Sum1/1 -> Mux6/3
  Constant9/1 -> Mux7/3, Mux7/1, Mux7/2
  Trigonometric Function8/1 -> Signal Specification4/1
  Trigonometric Function9/1 -> Signal Specification1/1
  Mux6/1 -> Trigonometric Function9/1, Trigonometric Function8/1
  Mux7/1 -> Matrix Concatenate2/3
  Matrix Concatenate2/1 -> Product/1

== system SG_GFOR_2020a_REAL/G1/Exciter System/PSS1 ==
  note: Power System Stabilizer (PSS2A)
  dw : Inport
  Pgen : Inport  Port=2
  Gain : Gain  Gain=Ks1
  Gain1 : Gain  Gain=Ks3
  Saturation : Saturate  UpperLimit=Vstmax  LowerLimit=Vstmin
  Sum1 : Sum  Inputs=|++
  Sum2 : Sum  Inputs=|+-
  Transfer Fcn1 : TransferFcn  Numerator=[Tw1 0]  Denominator=[Tw1 1]
  Transfer Fcn2 : TransferFcn  Numerator=[Tw3 0]  Denominator=[Tw3 1]
  Transfer Fcn3 : TransferFcn  Numerator=[Tw2 0]  Denominator=[Tw2 1]
  Transfer Fcn4 : TransferFcn  Denominator=[T6 1]
  Transfer Fcn5 : TransferFcn  Numerator=[T8 1].^N  Denominator=[T9 1].^(M*N)
  Transfer Fcn6 : TransferFcn  Numerator=[T1 1]  Denominator=[T2 1]
  Transfer Fcn7 : TransferFcn  Numerator=[T3 1]  Denominator=[T4 1]
  Transfer Fcn8 : TransferFcn  Numerator=[Tw4 0]  Denominator=[Tw4 1]
  Transfer Fcn9 : TransferFcn  Numerator=[Ks2]  Denominator=[T7 1]
  Vothsg : Outport
  wires:
  dw/1 -> Transfer Fcn1/1
  Transfer Fcn1/1 -> Transfer Fcn3/1
  Transfer Fcn3/1 -> Transfer Fcn4/1
  Transfer Fcn4/1 -> Sum1/1
  Sum1/1 -> Transfer Fcn5/1
  Transfer Fcn5/1 -> Sum2/1
  Sum2/1 -> Gain/1
  Gain/1 -> Transfer Fcn6/1
  Transfer Fcn6/1 -> Transfer Fcn7/1
  Transfer Fcn7/1 -> Saturation/1
  Saturation/1 -> Vothsg/1
  Pgen/1 -> Transfer Fcn2/1
  Transfer Fcn2/1 -> Transfer Fcn8/1
  Transfer Fcn8/1 -> Transfer Fcn9/1
  Gain1/1 -> Sum1/2
  Transfer Fcn9/1 -> Gain1/1, Sum2/2

== system SG_GFOR_2020a_REAL/G1/Exciter System/PSS1 backup ==
  note: Power System Stabilizer (PSS2A)
  dw : Inport
  Pgen : Inport  Port=2
  Gain : Gain  Gain=Ks1
  Gain1 : Gain  Gain=Ks3
  Saturation : Saturate  UpperLimit=Vstmax  LowerLimit=Vstmin
  Sum1 : Sum  Inputs=|++
  Sum2 : Sum  Inputs=|+-
  Transfer Fcn1 : TransferFcn  Numerator=[Tw1 0]  Denominator=[Tw1 1]
  Transfer Fcn2 : TransferFcn  Numerator=[Tw3 0]  Denominator=[Tw3 1]
  Transfer Fcn3 : TransferFcn  Numerator=[Tw2 0]  Denominator=[Tw2 1]
  Transfer Fcn4 : TransferFcn  Denominator=[T6 1]
  Transfer Fcn5 : TransferFcn  Numerator=[T8 1].^N  Denominator=[T9 1].^(M*N)
  Transfer Fcn6 : TransferFcn  Numerator=[T1 1]  Denominator=[T2 1]
  Transfer Fcn7 : TransferFcn  Numerator=[T3 1]  Denominator=[T4 1]
  Transfer Fcn8 : TransferFcn  Numerator=[Tw4 0]  Denominator=[Tw4 1]
  Transfer Fcn9 : TransferFcn  Numerator=[Ks2]  Denominator=[T7 1]
  Vothsg : Outport
  wires:
  Transfer Fcn9/1 -> Sum2/2, Gain1/1
  Gain1/1 -> Sum1/2
  Transfer Fcn8/1 -> Transfer Fcn9/1
  Transfer Fcn2/1 -> Transfer Fcn8/1
  Pgen/1 -> Transfer Fcn2/1
  Saturation/1 -> Vothsg/1
  Transfer Fcn7/1 -> Saturation/1
  Transfer Fcn6/1 -> Transfer Fcn7/1
  Gain/1 -> Transfer Fcn6/1
  Sum2/1 -> Gain/1
  Transfer Fcn5/1 -> Sum2/1
  Sum1/1 -> Transfer Fcn5/1
  Transfer Fcn4/1 -> Sum1/1
  Transfer Fcn3/1 -> Transfer Fcn4/1
  Transfer Fcn1/1 -> Transfer Fcn3/1
  dw/1 -> Transfer Fcn1/1

== system SG_GFOR_2020a_REAL/G1/Exciter System/SEXS ==
  note: The controller parameters provided by ENTSO-E
      | define different names for the parameters:
      |
      | ENTSO-E = IEEE Std 421.5-2005
      | Ta = Tc
      | Tb = Tb
      | K = Ka
      | Te = Ta
      | Emax = Vrmax
      | Emin = Vrmin
  note: The exciter model provided by ENTSO-E most similar to the IEEE is the Type AC4A excitation system model
  Vref : Inport
  Vc : Inport  Port=2
  Vs : Inport  Port=3
  1st ord transfer fcn windup limiter : Subsystem  mask{Gain=K, tau=Te, Vmax=Emax, Vmin=Emin, y0=Vf0}
      mask prompts: tau "Time constant"; y0 "Initial output"
  Constant : Constant  Value=Vf0/K
  Saturation : Saturate  Commented=through  UpperLimit=0.1  LowerLimit=-0.1
  Sum : Sum  Inputs=+-+
  Sum1 : Sum  Inputs=|++
  Transfer Fcn (with initial outputs)1 : simulink_extras/Additional Linear/Transfer Fcn (with initial outputs)  N=[Ta 1]  D=[Tb 1]  Y0=Vf0/K  U0=Vf0/K
  Efd : Outport
  wires:
  1st ord transfer fcn windup limiter/1(Out1) -> Efd/1
  Vs/1 -> Sum/3
  Vref/1 -> Sum/1
  Vc/1 -> Sum/2
  Transfer Fcn (with initial outputs)1/1 -> 1st ord transfer fcn windup limiter/1(In1)
  Saturation/1 -> Transfer Fcn (with initial outputs)1/1
  Sum/1 -> Sum1/1
  Sum1/1 -> Saturation/1
  Constant/1 -> Sum1/2

== system SG_GFOR_2020a_REAL/G1/Exciter System/TR and LC_test ==
  note: Terminal voltage transducer and optional load compensation
  note: compensated
      | impedance
  note: Vt and It should be phasors (complex quantities)
  note: Fig 4.1 of IEEE Std 421.5-2005
  note: Rc and Xc should be negative values in case of voltage regulated after an impedance
  Vt : Inport
  It : Inport  Port=2
  Abs : Abs
  Abs1 : Abs
  Rc+jXc : Gain  Gain=abs(Rc+1i*Xc)
  Saturation : Saturate  UpperLimit=1.2  LowerLimit=0.8
  Sum : Sum  Inputs=|+-
  Transfer Fcn (with initial outputs) : simulink_extras/Additional Linear/Transfer Fcn (with initial outputs)  Commented=through  N=[1]  D=[Tr 1]  Y0=1  U0=1
  Vc : Outport
  wires:
  Saturation/1 -> Vc/1
  Vt/1 -> Abs/1
  Transfer Fcn (with initial outputs)/1 -> Saturation/1
  Rc+jXc/1 -> Sum/2
  Sum/1 -> Transfer Fcn (with initial outputs)/1
  It/1 -> Abs1/1
  Abs/1 -> Sum/1
  Abs1/1 -> Rc+jXc/1

== system SG_GFOR_2020a_REAL/VSC/Current regulator/ParkInverse ==
  ABC vector : Inport
  angle : Inport  Port=2
  Constant4 : Constant  Value=2*pi/3
  Constant5 : Constant  Value=2*pi/3
  Constant9 : Constant
  Matrix Concatenate2 : Concatenate  NumInputs=3  Mode=Multidimensional array  ConcatenateDimension=2
  Mux6 : Mux  Inputs=3
  Mux7 : Mux  Inputs=3
  Product : Product  Multiplication=Matrix(*)  RndMeth=Zero
  Sum : Sum  Inputs=|+-
  Sum1 : Sum  Inputs=|++
  Trigonometric Function8 : Trigonometry  Operator=cos
  Trigonometric Function9 : Trigonometry
  Matrix : Outport
  wires:
  angle/1 -> Sum1/1, Sum/1, Mux6/1
  Constant5/1 -> Sum1/2
  Constant4/1 -> Sum/2
  Product/1 -> Matrix/1
  ABC vector/1 -> Product/2
  Sum/1 -> Mux6/2
  Sum1/1 -> Mux6/3
  Constant9/1 -> Mux7/3, Mux7/1, Mux7/2
  Trigonometric Function8/1 -> Matrix Concatenate2/1
  Trigonometric Function9/1 -> Matrix Concatenate2/2
  Mux6/1 -> Trigonometric Function9/1, Trigonometric Function8/1
  Mux7/1 -> Matrix Concatenate2/3
  Matrix Concatenate2/1 -> Product/1

== system SG_GFOR_2020a_REAL/Do not use/PQ/PLL/ParkTransform7 ==
  ABC vector : Inport
  angle : Inport  Port=2
  Constant1 : Constant  Value=1/2
  Constant2 : Constant  Value=1/2
  Constant3 : Constant  Value=2*pi/3
  Constant4 : Constant  Value=2*pi/3
  Constant5 : Constant  Value=1/2
  Gain : Gain  Gain=2/3
  Matrix Concatenate : Concatenate  NumInputs=3  Mode=Multidimensional array  ConcatenateDimension=2
  Mux1 : Mux  Inputs=3
  Mux2 : Mux  Inputs=3
  Mux3 : Mux  Inputs=3
  Product : Product  Multiplication=Matrix(*)  RndMeth=Zero
  Sum : Sum  Inputs=|+-
  Sum1 : Sum  Inputs=|++
  Trigonometric Function1 : Trigonometry  Operator=cos
  Trigonometric Function2 : Trigonometry  Operator=cos
  Trigonometric Function3 : Trigonometry
  Trigonometric Function4 : Trigonometry
  Trigonometric Function5 : Trigonometry  Operator=cos
  Trigonometric Function6 : Trigonometry
  Matrix : Outport
  wires:
  Mux3/1 -> Matrix Concatenate/3
  Mux2/1 -> Matrix Concatenate/1
  Mux1/1 -> Matrix Concatenate/2
  Sum1/1 -> Trigonometric Function5/1, Trigonometric Function6/1
  Constant5/1 -> Mux3/3
  Trigonometric Function5/1 -> Mux3/1
  Trigonometric Function6/1 -> Mux3/2
  Constant1/1 -> Mux2/3
  Trigonometric Function1/1 -> Mux2/1
  Trigonometric Function4/1 -> Mux2/2
  Sum/1 -> Trigonometric Function2/1, Trigonometric Function3/1
  Constant2/1 -> Mux1/3
  Trigonometric Function2/1 -> Mux1/1
  Trigonometric Function3/1 -> Mux1/2
  angle/1 -> Sum/1, Sum1/1, Trigonometric Function1/1, Trigonometric Function4/1
  Constant3/1 -> Sum1/2
  Constant4/1 -> Sum/2
  Gain/1 -> Product/1
  Product/1 -> Matrix/1
  ABC vector/1 -> Product/2
  Matrix Concatenate/1 -> Gain/1

== system SG_GFOR_2020a_REAL/G1/Exciter System/SEXS/1st ord transfer fcn windup limiter ==
  note: First order transfer function with windup limiter (non-saturated output)
  In1 : Inport
  Compare To Constant : simulink/Logic and Bit Operations/Compare To Constant  relop=<=  const=Vmax  OutDataTypeStr=boolean
  Compare To Constant1 : simulink/Logic and Bit Operations/Compare To Constant  relop=>=  const=Vmin  OutDataTypeStr=boolean
  OR : Logic  Operator=OR  IconShape=distinctive  AllPortsSameDT=off  OutDataTypeStr=boolean
  Sample and Hold1 : powerlib_meascontrol/Additional Components/Sample and Hold  ic=0  Ts=0
      settings: SourceProductBaseCode=PS
  Saturation1 : Saturate  UpperLimit=Vmax  LowerLimit=Vmin
  Transfer Fcn (with initial outputs)2 : simulink_extras/Additional Linear/Transfer Fcn (with initial outputs)  N=[Gain]  D=[tau 1]  Y0=y0  U0=y0/Gain
  Out1 : Outport
  wires:
  Sample and Hold1/1 -> Transfer Fcn (with initial outputs)2/1
  Transfer Fcn (with initial outputs)2/1 -> Saturation1/1, Compare To Constant1/1, Compare To Constant/1
  In1/1 -> Sample and Hold1/1
  Compare To Constant/1 -> OR/1
  Compare To Constant1/1 -> OR/2
  OR/1 -> Sample and Hold1/2
  Saturation1/1 -> Out1/1
